simulink model "SSN_39busRT_Ctrl_4WT_19B"  (R2021a)
settings: Solver=ode3  StartTime=0.0  StopTime=10  FixedStep=Ts  MaxStep=1/60  RelTol=1e-2  AbsTol=1e-1
PreLoadFcn:
  | Ts=2.50e-6; ssn_ieee39_params; load('Pwf.mat');
InitFcn:
  | Ts=2.50e-6; ssn_ieee39_params; load('Pwf.mat');
values from neighbouring files (symbols this model uses):
  f = 50    [ssn_ieee39_params_ctrl.m]
  fNom = f    (= 60)    [ssn_ieee39_params_ctrl.m]
  ILR = 5.02    [ssn_ieee39_params_ctrl.m]
  IQMIN = 0.1    [ssn_ieee39_params_ctrl.m]
  ISCLIM = 1    [ssn_ieee39_params_ctrl.m]
  ITFpu = 1.10    (= 1.1)    [ssn_ieee39_params_ctrl.m]
  K = 1    [ssn_ieee39_params_ctrl.m]
  K1 = 1    [ssn_ieee39_params_ctrl.m]
  K2 = 2    [ssn_ieee39_params_ctrl.m]
  KCL = 1.04    [ssn_ieee39_params_ctrl.m]
  KFB = 0    [ssn_ieee39_params_ctrl.m]
  KFF = 1    [ssn_ieee39_params_ctrl.m]
  KFIX = 1    [ssn_ieee39_params_ctrl.m]
  KG = 1    [ssn_ieee39_params_ctrl.m]
  KIA = 59.91    [ssn_ieee39_params_ctrl.m]
  KIOEX = 0.0303    [ssn_ieee39_params_ctrl.m]
  KIUEX = 0.0303    [ssn_ieee39_params_ctrl.m]
  KIUOEX = 1    [ssn_ieee39_params_ctrl.m]
  KIUUEX = 1    [ssn_ieee39_params_ctrl.m]
  KLR = 22.47    [ssn_ieee39_params_ctrl.m]
  KM = 1    [ssn_ieee39_params_ctrl.m]
  KOEL = 0.24    [ssn_ieee39_params_ctrl.m]
  Kp = 1    [ssn_ieee39_params_ctrl.m]
  KPA = 30    [ssn_ieee39_params_ctrl.m]
  KPOEL = 1    [ssn_ieee39_params_ctrl.m]
  KPOEX = 0    [ssn_ieee39_params_ctrl.m]
  KPUEX = 0    [ssn_ieee39_params_ctrl.m]
  KSCALE = 0.319    [ssn_ieee39_params_ctrl.m]
  KUF = 0    [ssn_ieee39_params_ctrl.m]
  KUI = 0.001    [ssn_ieee39_params_ctrl.m]
  KUL = 0.24    [ssn_ieee39_params_ctrl.m]
  s = 10    [ssn_ieee39_params_ctrl.m]
  TA = 0.01    [ssn_ieee39_params_ctrl.m]
  Tadj = 0    [ssn_ieee39_params_ctrl.m]
  taps = [1 1 1.07 1.07 1.009 1.025 1 1.025 1.025 1.025]*1    [ssn_ieee39_params_ctrl.m]
  TF = 0.02    [ssn_ieee39_params_ctrl.m]
  TG = 0.024    [ssn_ieee39_params_ctrl.m]
  TINV = 0    [ssn_ieee39_params_ctrl.m]
  TIT = 0.1    [ssn_ieee39_params_ctrl.m]
  TL_10_11_len = 14    [ssn_ieee39_params_ctrl.m]
  TL_10_13_len = 14    [ssn_ieee39_params_ctrl.m]
  TL_13_14_len = 32    [ssn_ieee39_params_ctrl.m]
  TL_14_15_len = 70    [ssn_ieee39_params_ctrl.m]
  TL_15_16_len = 31.5    [ssn_ieee39_params_ctrl.m]
  TL_16_17_len = 26    [ssn_ieee39_params_ctrl.m]
  TL_16_19_len = 61    [ssn_ieee39_params_ctrl.m]
  TL_16_21_len = 46    [ssn_ieee39_params_ctrl.m]
  TL_16_24_len = 15    [ssn_ieee39_params_ctrl.m]
  TL_17_18_len = 26    [ssn_ieee39_params_ctrl.m]
  TL_17_27_len = 59    [ssn_ieee39_params_ctrl.m]
  TL_1_2_len = 134    [ssn_ieee39_params_ctrl.m]
  TL_1_39_len = 105    [ssn_ieee39_params_ctrl.m]
  TL_21_22_len = 47    [ssn_ieee39_params_ctrl.m]
  TL_22_23_len = 33    [ssn_ieee39_params_ctrl.m]
  TL_24_23_len = 88    [ssn_ieee39_params_ctrl.m]
  TL_25_26_len = 101    [ssn_ieee39_params_ctrl.m]
  TL_26_27_len = 46.5    [ssn_ieee39_params_ctrl.m]
  TL_26_28_len = 151    [ssn_ieee39_params_ctrl.m]
  TL_26_29_len = 200    [ssn_ieee39_params_ctrl.m]
  TL_28_29_len = 48    [ssn_ieee39_params_ctrl.m]
  TL_2_25_len = 28    [ssn_ieee39_params_ctrl.m]
  TL_2_2_len = 49    [ssn_ieee39_params_ctrl.m]
  TL_3_18_len = 42    [ssn_ieee39_params_ctrl.m]
  TL_3_4_len = 53    [ssn_ieee39_params_ctrl.m]
  TL_4_14_len = 33    [ssn_ieee39_params_ctrl.m]
  TL_4_5_len = 32.5    [ssn_ieee39_params_ctrl.m]
  TL_5_6_len = 14    [ssn_ieee39_params_ctrl.m]
  TL_5_8_len = 32    [ssn_ieee39_params_ctrl.m]
  TL_6_11_len = 26.5    [ssn_ieee39_params_ctrl.m]
  TL_6_7_len = 25.5    [ssn_ieee39_params_ctrl.m]
  TL_7_8_len = 15    [ssn_ieee39_params_ctrl.m]
  TL_8_9_len = 93    [ssn_ieee39_params_ctrl.m]
  TL_9_39_len = 136    [ssn_ieee39_params_ctrl.m]
  TOEL = 5.00    (= 5)    [ssn_ieee39_params_ctrl.m]
  TQREF = 0    [ssn_ieee39_params_ctrl.m]
  TQSCL = 0.012    [ssn_ieee39_params_ctrl.m]
  Ts_PMU = 1/1000    (= 0.001)    [ssn_ieee39_params_ctrl.m]
  TU1 = 0    [ssn_ieee39_params_ctrl.m]
  TU2 = 0    [ssn_ieee39_params_ctrl.m]
  TU3 = 0    [ssn_ieee39_params_ctrl.m]
  TU4 = 0    [ssn_ieee39_params_ctrl.m]
  TUL = 0    [ssn_ieee39_params_ctrl.m]
  TUP = 0.050    (= 0.05)    [ssn_ieee39_params_ctrl.m]
  TUQ = .005    (= 0.005)    [ssn_ieee39_params_ctrl.m]
  TUV = 0.2    [ssn_ieee39_params_ctrl.m]
  VAAMAX = VAMAX    (= 7.05)    [ssn_ieee39_params_ctrl.m]
  VAMAX = 7.05    [ssn_ieee39_params_ctrl.m]
  VAMIN = -6.11    [ssn_ieee39_params_ctrl.m]
  VBMAX = 999    [ssn_ieee39_params_ctrl.m]
  VF = 0    [ssn_ieee39_params_ctrl.m]
  VFB = 0    [ssn_ieee39_params_ctrl.m]
  VMMAX = 7.05    [ssn_ieee39_params_ctrl.m]
  VMMIN = -6.11    [ssn_ieee39_params_ctrl.m]
  VOELmax1 = 0.2353    [ssn_ieee39_params_ctrl.m]
  VOELmax2 = 0.0    (= 0)    [ssn_ieee39_params_ctrl.m]
  VOELmin1 = -0.24    [ssn_ieee39_params_ctrl.m]
  VOELmin2 = -1.0    (= -1)    [ssn_ieee39_params_ctrl.m]
  VRMAX = 7.05    [ssn_ieee39_params_ctrl.m]
  VRMIN = -6.11    [ssn_ieee39_params_ctrl.m]
  VSCLmax = 0.20    (= 0.2)    [ssn_ieee39_params_ctrl.m]
  VSCLmin = -0.10    (= -0.1)    [ssn_ieee39_params_ctrl.m]
  VUELmax1 = 1    [ssn_ieee39_params_ctrl.m]
  VUELmax2 = 1    [ssn_ieee39_params_ctrl.m]
  VUELmin1 = -1    [ssn_ieee39_params_ctrl.m]
  VUELmin2 = -1    [ssn_ieee39_params_ctrl.m]
  VUImax = 1    [ssn_ieee39_params_ctrl.m]
  VUImin = -1    [ssn_ieee39_params_ctrl.m]
undefined symbols (not defined in the file or in its folder): another_event_name, D1, Delta, DiscIntNeverNeededParam, find_system, MOV_segment9, my_event_name, powergui, Pw1, Pw2, Pw3, Pw4, vNomHV
libraries: powerlib_extras x162, spsThreePhaseVIMeasurementLib x55, spsCurrentMeasurementLib x52, simulink_extras x44, slpidlib x40, op_dpl_lib x36, spsST2AModel x20, spsThreePhaseParallelRLCLoadLib x20, spsThreePhaseTransformerTwoWindingsLib x17, spsControlledVoltageSourceLib x16, spsVoltageMeasurementLib x12, spsSynchronousMachinepuStandardLib x10
(part 19 of 19)

== system SSN_39busRT_Ctrl_4WT_19B/SM_master/4 WT/SS_windfarm1to2/Wind Farm (DFIG Type)/Wind Turbine Doubly-Fed Induction Generator (Average Model)1/Control System_average/Control/Rotor-side converter Control system/Torque control/Torque reference/Looses ==
  wr : Inport
  Idqs : Inport  Port=2
  Idq_grid_conv : Inport  Port=3
  Idqr : Inport  Port=4
  Freq : Inport  Port=5
  Constant3 : Constant  Value=R_RL
  Discrete Variable Frequency Mean value : Subsystem  mask(Discrete Variable-Frequency Mean Value){Finit=Fnom, Fmin=45, Ts=Ts_Control}
      mask prompts: Finit "Initial frequency (Hz):"; Fmin "Minimum frequency (Hz):"; Ts "Sample time:"
      mask help:
      | This discrete block computes the mean value of the input signal (port In) over a running window of one cycle of a specified frequency (port Freq).
      |
      | For the first cycle of simulation (specified by the parameter "Initial frequency"), the ouput is held to the value of the  "Initial input" parameter.
      |
      | The value of the parameter "Minimum frequency" is used to determine the buffer size of the "Variable Transport Delay" block found inside this subsystem.
      mask init:
      | MaxDelay=1/Fmin+Ts;
  Friction Factor : Gain  Gain=F  SaturateOnIntegerOverflow=on  OutDataTypeStr=Inherit: Same as input  ParamDataTypeStr=Inherit: Same as input
  Product{1..4} (4 alike) : Product  InputSameDT=on  SaturateOnIntegerOverflow=on  OutDataTypeStr=Inherit: Same as first input
  Rr : Constant  Value=Rr
  Rs : Constant  Value=Rs
  Sum2 : Sum  Inputs=+++  SaturateOnIntegerOverflow=on
  Sum5 : Sum  Inputs=|++  SaturateOnIntegerOverflow=on
  id^2+iq^2 : Fcn  Expr=u(1)^2+u(2)^2
  "id^2+iq^2 " : Fcn  Expr=u(1)^2+u(2)^2
  "id^2+iq^2   " : Fcn  Expr=u(1)^2+u(2)^2
  P_looses : Outport
  wires:
  Idqr/1 -> "id^2+iq^2 "/1
  Idqs/1 -> id^2+iq^2/1
  Discrete Variable Frequency Mean value/1(Mean) -> P_looses/1
  Sum5/1 -> Sum2/3
  Product1/1 -> Sum5/2
  Product4/1 -> Sum5/1
  Idq_grid_conv/1 -> "id^2+iq^2   "/1
  "id^2+iq^2   "/1 -> Product1/2
  Constant3/1 -> Product1/1
  wr/1 -> Product2/1, Friction Factor/1
  Sum2/1 -> Discrete Variable Frequency Mean value/2(In), Discrete Variable Frequency Mean value/3(Init)  "Looses"
  Product2/1 -> Sum2/1
  Product3/1 -> Sum2/2
  "id^2+iq^2 "/1 -> Product4/2
  Rr/1 -> Product4/1
  id^2+iq^2/1 -> Product3/2
  Rs/1 -> Product3/1
  Friction Factor/1 -> Product2/2  "T_Friction"
  Freq/1 -> Discrete Variable Frequency Mean value/1(Freq)

== system SSN_39busRT_Ctrl_4WT_19B/SM_master/4 WT/SS_windfarm1to2/Wind Farm (DFIG Type)/Wind Turbine Doubly-Fed Induction Generator (Average Model)1/Control System_average/Control/Rotor-side converter Control system/Torque control/Torque reference/Slope_B_A ==
  Constant6 : Constant  Value=power_B
  Constant7 : Constant  Value=power_A
  Constant8 : Constant  Value=speed_B
  Constant9 : Constant  Value=speed_A
  Product2 : Product  Inputs=*/  SaturateOnIntegerOverflow=on  OutDataTypeStr=Inherit: Same as first input
  Sum8 : Sum  Inputs=|+-  SaturateOnIntegerOverflow=on
  Sum9 : Sum  Inputs=|+-  SaturateOnIntegerOverflow=on
  Slope : Outport
  wires:
  Constant6/1 -> Sum8/1
  Constant7/1 -> Sum8/2
  Constant8/1 -> Sum9/1
  Constant9/1 -> Sum9/2
  Sum8/1 -> Product2/1
  Sum9/1 -> Product2/2
  Product2/1 -> Slope/1

== system SSN_39busRT_Ctrl_4WT_19B/SM_master/4 WT/SS_windfarm1to2/Wind Farm (DFIG Type)/Wind Turbine Doubly-Fed Induction Generator (Average Model)1/Control System_average/Control/Rotor-side converter Control system/Torque control/Torque reference/Slope_D_C ==
  Constant2 : Constant  Value=power_D
  Constant3 : Constant  Value=power_C
  Constant4 : Constant  Value=speed_D
  Constant5 : Constant  Value=speed_C
  Product : Product  Inputs=*/  SaturateOnIntegerOverflow=on  OutDataTypeStr=Inherit: Same as first input
  Sum6 : Sum  Inputs=|+-  SaturateOnIntegerOverflow=on
  Sum7 : Sum  Inputs=|+-  SaturateOnIntegerOverflow=on
  Slope : Outport
  wires:
  Constant2/1 -> Sum6/1
  Constant3/1 -> Sum6/2
  Constant4/1 -> Sum7/1
  Constant5/1 -> Sum7/2
  Sum6/1 -> Product/1
  Sum7/1 -> Product/2
  Product/1 -> Slope/1

== system SSN_39busRT_Ctrl_4WT_19B/SM_master/4 WT/SS_windfarm1to2/Wind Farm (DFIG Type)/Wind Turbine Doubly-Fed Induction Generator (Average Model)1/Control System_average/Control/Rotor-side converter Control system/Torque control/Torque regulator/Stator flux estimator ==
  note: Magnitude of flux at generator stator
      | The derivative components of flux are neglected
  Vdqs : Inport
  Idqs : Inport  Port=2
  Freq : Inport  Port=3
  Divide1 : Product  Inputs=*/
  Divide2 : Product  Inputs=**
  Divide3 : Product  Inputs=*/
  Divide4 : Product  Inputs=*/
  Divide6 : Product  Inputs=**
  Fnom : Constant  Value=Fnom
  Gain : Gain  Gain=-1
  Math Function1 : Math  Operator=square  SignedPower=on  SaturateOnIntegerOverflow=on
  Math Function2 : Math  Operator=square  SignedPower=on  SaturateOnIntegerOverflow=on
  Math Function3 : Math  Operator=sqrt  SignedPower=on  SaturateOnIntegerOverflow=on
  Rs : Constant  Value=Rs
  Rs2 : Constant  Value=Rs
  Selector1 : Selector  InputPortWidth=2  IndexOptions=Index vector (dialog)  Indices=2  OutputSizes=[(-2)]
  Selector2 : Selector  InputPortWidth=2  IndexOptions=Index vector (dialog)  Indices=1  OutputSizes=[(-2)]
  Selector3 : Selector  InputPortWidth=2  IndexOptions=Index vector (dialog)  Indices=2  OutputSizes=[(-2)]
  Selector4 : Selector  InputPortWidth=2  IndexOptions=Index vector (dialog)  Indices=1  OutputSizes=[(-2)]
  Sum1 : Sum  Inputs=|++
  Sum2 : Sum  Inputs=|+-
  Sum3 : Sum  Inputs=|+-
  Mag_Flux : Outport
  wires:
  Math Function2/1 -> Sum1/2
  Divide4/1 -> Math Function2/1  "phi_ds"
  Sum2/1 -> Divide4/1
  Divide2/1 -> Sum2/2  "RsIqs"
  Rs2/1 -> Divide2/2
  Selector3/1 -> Divide2/1  "Iqs"
  Selector1/1 -> Sum2/1  "Vqs"
  Math Function3/1 -> Mag_Flux/1
  Sum1/1 -> Math Function3/1
  Math Function1/1 -> Sum1/1
  Divide1/1 -> Math Function1/1  "phi_qs"
  Gain/1 -> Divide1/2
  Divide3/1 -> Divide4/2, Gain/1
  Sum3/1 -> Divide1/1
  Fnom/1 -> Divide3/2
  Freq/1 -> Divide3/1
  Selector4/1 -> Sum3/1  "Vds"
  Vdqs/1 -> Selector1/1, Selector4/1
  Rs/1 -> Divide6/2
  Selector2/1 -> Divide6/1  "Ids"
  Divide6/1 -> Sum3/2  "RsIds"
  Idqs/1 -> Selector3/1, Selector2/1

== system SSN_39busRT_Ctrl_4WT_19B/SM_master/4 WT/SS_windfarm1to2/Wind Farm (DFIG Type)1/Wind Turbine Doubly-Fed Induction Generator (Average Model)1/Control System_average/Control/Rotor-side converter Control system/Torque control/Torque reference/Looses ==
  wr : Inport
  Idqs : Inport  Port=2
  Idq_grid_conv : Inport  Port=3
  Idqr : Inport  Port=4
  Freq : Inport  Port=5
  Constant3 : Constant  Value=R_RL
  Discrete Variable Frequency Mean value : Subsystem  mask(Discrete Variable-Frequency Mean Value){Finit=Fnom, Fmin=45, Ts=Ts_Control}
      mask prompts: Finit "Initial frequency (Hz):"; Fmin "Minimum frequency (Hz):"; Ts "Sample time:"
      mask help:
      | This discrete block computes the mean value of the input signal (port In) over a running window of one cycle of a specified frequency (port Freq).
      |
      | For the first cycle of simulation (specified by the parameter "Initial frequency"), the ouput is held to the value of the  "Initial input" parameter.
      |
      | The value of the parameter "Minimum frequency" is used to determine the buffer size of the "Variable Transport Delay" block found inside this subsystem.
      mask init:
      | MaxDelay=1/Fmin+Ts;
  Friction Factor : Gain  Gain=F  SaturateOnIntegerOverflow=on  OutDataTypeStr=Inherit: Same as input  ParamDataTypeStr=Inherit: Same as input
  Product{1..4} (4 alike) : Product  InputSameDT=on  SaturateOnIntegerOverflow=on  OutDataTypeStr=Inherit: Same as first input
  Rr : Constant  Value=Rr
  Rs : Constant  Value=Rs
  Sum2 : Sum  Inputs=+++  SaturateOnIntegerOverflow=on
  Sum5 : Sum  Inputs=|++  SaturateOnIntegerOverflow=on
  id^2+iq^2 : Fcn  Expr=u(1)^2+u(2)^2
  "id^2+iq^2 " : Fcn  Expr=u(1)^2+u(2)^2
  "id^2+iq^2   " : Fcn  Expr=u(1)^2+u(2)^2
  P_looses : Outport
  wires:
  Freq/1 -> Discrete Variable Frequency Mean value/1(Freq)
  Friction Factor/1 -> Product2/2  "T_Friction"
  Rs/1 -> Product3/1
  id^2+iq^2/1 -> Product3/2
  Rr/1 -> Product4/1
  "id^2+iq^2 "/1 -> Product4/2
  Product3/1 -> Sum2/2
  Product2/1 -> Sum2/1
  Sum2/1 -> Discrete Variable Frequency Mean value/3(Init), Discrete Variable Frequency Mean value/2(In)  "Looses"
  wr/1 -> Friction Factor/1, Product2/1
  Constant3/1 -> Product1/1
  "id^2+iq^2   "/1 -> Product1/2
  Idq_grid_conv/1 -> "id^2+iq^2   "/1
  Product4/1 -> Sum5/1
  Product1/1 -> Sum5/2
  Sum5/1 -> Sum2/3
  Discrete Variable Frequency Mean value/1(Mean) -> P_looses/1
  Idqs/1 -> id^2+iq^2/1
  Idqr/1 -> "id^2+iq^2 "/1

== system SSN_39busRT_Ctrl_4WT_19B/SM_master/4 WT/SS_windfarm1to2/Wind Farm (DFIG Type)1/Wind Turbine Doubly-Fed Induction Generator (Average Model)1/Control System_average/Control/Rotor-side converter Control system/Torque control/Torque reference/Slope_B_A ==
  Constant6 : Constant  Value=power_B
  Constant7 : Constant  Value=power_A
  Constant8 : Constant  Value=speed_B
  Constant9 : Constant  Value=speed_A
  Product2 : Product  Inputs=*/  SaturateOnIntegerOverflow=on  OutDataTypeStr=Inherit: Same as first input
  Sum8 : Sum  Inputs=|+-  SaturateOnIntegerOverflow=on
  Sum9 : Sum  Inputs=|+-  SaturateOnIntegerOverflow=on
  Slope : Outport
  wires:
  Product2/1 -> Slope/1
  Sum9/1 -> Product2/2
  Sum8/1 -> Product2/1
  Constant9/1 -> Sum9/2
  Constant8/1 -> Sum9/1
  Constant7/1 -> Sum8/2
  Constant6/1 -> Sum8/1

== system SSN_39busRT_Ctrl_4WT_19B/SM_master/4 WT/SS_windfarm1to2/Wind Farm (DFIG Type)1/Wind Turbine Doubly-Fed Induction Generator (Average Model)1/Control System_average/Control/Rotor-side converter Control system/Torque control/Torque reference/Slope_D_C ==
  Constant2 : Constant  Value=power_D
  Constant3 : Constant  Value=power_C
  Constant4 : Constant  Value=speed_D
  Constant5 : Constant  Value=speed_C
  Product : Product  Inputs=*/  SaturateOnIntegerOverflow=on  OutDataTypeStr=Inherit: Same as first input
  Sum6 : Sum  Inputs=|+-  SaturateOnIntegerOverflow=on
  Sum7 : Sum  Inputs=|+-  SaturateOnIntegerOverflow=on
  Slope : Outport
  wires:
  Product/1 -> Slope/1
  Sum7/1 -> Product/2
  Sum6/1 -> Product/1
  Constant5/1 -> Sum7/2
  Constant4/1 -> Sum7/1
  Constant3/1 -> Sum6/2
  Constant2/1 -> Sum6/1

== system SSN_39busRT_Ctrl_4WT_19B/SM_master/4 WT/SS_windfarm1to2/Wind Farm (DFIG Type)1/Wind Turbine Doubly-Fed Induction Generator (Average Model)1/Control System_average/Control/Rotor-side converter Control system/Torque control/Torque regulator/Stator flux estimator ==
  note: Magnitude of flux at generator stator
      | The derivative components of flux are neglected
  Vdqs : Inport
  Idqs : Inport  Port=2
  Freq : Inport  Port=3
  Divide1 : Product  Inputs=*/
  Divide2 : Product  Inputs=**
  Divide3 : Product  Inputs=*/
  Divide4 : Product  Inputs=*/
  Divide6 : Product  Inputs=**
  Fnom : Constant  Value=Fnom
  Gain : Gain  Gain=-1
  Math Function1 : Math  Operator=square  SignedPower=on  SaturateOnIntegerOverflow=on
  Math Function2 : Math  Operator=square  SignedPower=on  SaturateOnIntegerOverflow=on
  Math Function3 : Math  Operator=sqrt  SignedPower=on  SaturateOnIntegerOverflow=on
  Rs : Constant  Value=Rs
  Rs2 : Constant  Value=Rs
  Selector1 : Selector  InputPortWidth=2  IndexOptions=Index vector (dialog)  Indices=2  OutputSizes=[(-2)]
  Selector2 : Selector  InputPortWidth=2  IndexOptions=Index vector (dialog)  Indices=1  OutputSizes=[(-2)]
  Selector3 : Selector  InputPortWidth=2  IndexOptions=Index vector (dialog)  Indices=2  OutputSizes=[(-2)]
  Selector4 : Selector  InputPortWidth=2  IndexOptions=Index vector (dialog)  Indices=1  OutputSizes=[(-2)]
  Sum1 : Sum  Inputs=|++
  Sum2 : Sum  Inputs=|+-
  Sum3 : Sum  Inputs=|+-
  Mag_Flux : Outport
  wires:
  Idqs/1 -> Selector2/1, Selector3/1
  Divide6/1 -> Sum3/2  "RsIds"
  Selector2/1 -> Divide6/1  "Ids"
  Rs/1 -> Divide6/2
  Vdqs/1 -> Selector4/1, Selector1/1
  Selector4/1 -> Sum3/1  "Vds"
  Freq/1 -> Divide3/1
  Fnom/1 -> Divide3/2
  Sum3/1 -> Divide1/1
  Divide3/1 -> Gain/1, Divide4/2
  Gain/1 -> Divide1/2
  Divide1/1 -> Math Function1/1  "phi_qs"
  Math Function1/1 -> Sum1/1
  Sum1/1 -> Math Function3/1
  Math Function3/1 -> Mag_Flux/1
  Selector1/1 -> Sum2/1  "Vqs"
  Selector3/1 -> Divide2/1  "Iqs"
  Rs2/1 -> Divide2/2
  Divide2/1 -> Sum2/2  "RsIqs"
  Sum2/1 -> Divide4/1
  Divide4/1 -> Math Function2/1  "phi_ds"
  Math Function2/1 -> Sum1/2

== system SSN_39busRT_Ctrl_4WT_19B/SM_master/4 WT/SS_windfarm3to4/Wind Farm (DFIG Type)/Wind Turbine Doubly-Fed Induction Generator (Average Model)1/Control System_average/Control/Rotor-side converter Control system/Torque control/Torque reference/Looses ==
  wr : Inport
  Idqs : Inport  Port=2
  Idq_grid_conv : Inport  Port=3
  Idqr : Inport  Port=4
  Freq : Inport  Port=5
  Constant3 : Constant  Value=R_RL
  Discrete Variable Frequency Mean value : Subsystem  mask(Discrete Variable-Frequency Mean Value){Finit=Fnom, Fmin=45, Ts=Ts_Control}
      mask prompts: Finit "Initial frequency (Hz):"; Fmin "Minimum frequency (Hz):"; Ts "Sample time:"
      mask help:
      | This discrete block computes the mean value of the input signal (port In) over a running window of one cycle of a specified frequency (port Freq).
      |
      | For the first cycle of simulation (specified by the parameter "Initial frequency"), the ouput is held to the value of the  "Initial input" parameter.
      |
      | The value of the parameter "Minimum frequency" is used to determine the buffer size of the "Variable Transport Delay" block found inside this subsystem.
      mask init:
      | MaxDelay=1/Fmin+Ts;
  Friction Factor : Gain  Gain=F  SaturateOnIntegerOverflow=on  OutDataTypeStr=Inherit: Same as input  ParamDataTypeStr=Inherit: Same as input
  Product{1..4} (4 alike) : Product  InputSameDT=on  SaturateOnIntegerOverflow=on  OutDataTypeStr=Inherit: Same as first input
  Rr : Constant  Value=Rr
  Rs : Constant  Value=Rs
  Sum2 : Sum  Inputs=+++  SaturateOnIntegerOverflow=on
  Sum5 : Sum  Inputs=|++  SaturateOnIntegerOverflow=on
  id^2+iq^2 : Fcn  Expr=u(1)^2+u(2)^2
  "id^2+iq^2 " : Fcn  Expr=u(1)^2+u(2)^2
  "id^2+iq^2   " : Fcn  Expr=u(1)^2+u(2)^2
  P_looses : Outport
  wires:
  Idqr/1 -> "id^2+iq^2 "/1
  Idqs/1 -> id^2+iq^2/1
  Discrete Variable Frequency Mean value/1(Mean) -> P_looses/1
  Sum5/1 -> Sum2/3
  Product1/1 -> Sum5/2
  Product4/1 -> Sum5/1
  Idq_grid_conv/1 -> "id^2+iq^2   "/1
  "id^2+iq^2   "/1 -> Product1/2
  Constant3/1 -> Product1/1
  wr/1 -> Product2/1, Friction Factor/1
  Sum2/1 -> Discrete Variable Frequency Mean value/2(In), Discrete Variable Frequency Mean value/3(Init)  "Looses"
  Product2/1 -> Sum2/1
  Product3/1 -> Sum2/2
  "id^2+iq^2 "/1 -> Product4/2
  Rr/1 -> Product4/1
  id^2+iq^2/1 -> Product3/2
  Rs/1 -> Product3/1
  Friction Factor/1 -> Product2/2  "T_Friction"
  Freq/1 -> Discrete Variable Frequency Mean value/1(Freq)

== system SSN_39busRT_Ctrl_4WT_19B/SM_master/4 WT/SS_windfarm3to4/Wind Farm (DFIG Type)/Wind Turbine Doubly-Fed Induction Generator (Average Model)1/Control System_average/Control/Rotor-side converter Control system/Torque control/Torque reference/Slope_B_A ==
  Constant6 : Constant  Value=power_B
  Constant7 : Constant  Value=power_A
  Constant8 : Constant  Value=speed_B
  Constant9 : Constant  Value=speed_A
  Product2 : Product  Inputs=*/  SaturateOnIntegerOverflow=on  OutDataTypeStr=Inherit: Same as first input
  Sum8 : Sum  Inputs=|+-  SaturateOnIntegerOverflow=on
  Sum9 : Sum  Inputs=|+-  SaturateOnIntegerOverflow=on
  Slope : Outport
  wires:
  Constant6/1 -> Sum8/1
  Constant7/1 -> Sum8/2
  Constant8/1 -> Sum9/1
  Constant9/1 -> Sum9/2
  Sum8/1 -> Product2/1
  Sum9/1 -> Product2/2
  Product2/1 -> Slope/1

== system SSN_39busRT_Ctrl_4WT_19B/SM_master/4 WT/SS_windfarm3to4/Wind Farm (DFIG Type)/Wind Turbine Doubly-Fed Induction Generator (Average Model)1/Control System_average/Control/Rotor-side converter Control system/Torque control/Torque reference/Slope_D_C ==
  Constant2 : Constant  Value=power_D
  Constant3 : Constant  Value=power_C
  Constant4 : Constant  Value=speed_D
  Constant5 : Constant  Value=speed_C
  Product : Product  Inputs=*/  SaturateOnIntegerOverflow=on  OutDataTypeStr=Inherit: Same as first input
  Sum6 : Sum  Inputs=|+-  SaturateOnIntegerOverflow=on
  Sum7 : Sum  Inputs=|+-  SaturateOnIntegerOverflow=on
  Slope : Outport
  wires:
  Constant2/1 -> Sum6/1
  Constant3/1 -> Sum6/2
  Constant4/1 -> Sum7/1
  Constant5/1 -> Sum7/2
  Sum6/1 -> Product/1
  Sum7/1 -> Product/2
  Product/1 -> Slope/1

== system SSN_39busRT_Ctrl_4WT_19B/SM_master/4 WT/SS_windfarm3to4/Wind Farm (DFIG Type)/Wind Turbine Doubly-Fed Induction Generator (Average Model)1/Control System_average/Control/Rotor-side converter Control system/Torque control/Torque regulator/Stator flux estimator ==
  note: Magnitude of flux at generator stator
      | The derivative components of flux are neglected
  Vdqs : Inport
  Idqs : Inport  Port=2
  Freq : Inport  Port=3
  Divide1 : Product  Inputs=*/
  Divide2 : Product  Inputs=**
  Divide3 : Product  Inputs=*/
  Divide4 : Product  Inputs=*/
  Divide6 : Product  Inputs=**
  Fnom : Constant  Value=Fnom
  Gain : Gain  Gain=-1
  Math Function1 : Math  Operator=square  SignedPower=on  SaturateOnIntegerOverflow=on
  Math Function2 : Math  Operator=square  SignedPower=on  SaturateOnIntegerOverflow=on
  Math Function3 : Math  Operator=sqrt  SignedPower=on  SaturateOnIntegerOverflow=on
  Rs : Constant  Value=Rs
  Rs2 : Constant  Value=Rs
  Selector1 : Selector  InputPortWidth=2  IndexOptions=Index vector (dialog)  Indices=2  OutputSizes=[(-2)]
  Selector2 : Selector  InputPortWidth=2  IndexOptions=Index vector (dialog)  Indices=1  OutputSizes=[(-2)]
  Selector3 : Selector  InputPortWidth=2  IndexOptions=Index vector (dialog)  Indices=2  OutputSizes=[(-2)]
  Selector4 : Selector  InputPortWidth=2  IndexOptions=Index vector (dialog)  Indices=1  OutputSizes=[(-2)]
  Sum1 : Sum  Inputs=|++
  Sum2 : Sum  Inputs=|+-
  Sum3 : Sum  Inputs=|+-
  Mag_Flux : Outport
  wires:
  Math Function2/1 -> Sum1/2
  Divide4/1 -> Math Function2/1  "phi_ds"
  Sum2/1 -> Divide4/1
  Divide2/1 -> Sum2/2  "RsIqs"
  Rs2/1 -> Divide2/2
  Selector3/1 -> Divide2/1  "Iqs"
  Selector1/1 -> Sum2/1  "Vqs"
  Math Function3/1 -> Mag_Flux/1
  Sum1/1 -> Math Function3/1
  Math Function1/1 -> Sum1/1
  Divide1/1 -> Math Function1/1  "phi_qs"
  Gain/1 -> Divide1/2
  Divide3/1 -> Divide4/2, Gain/1
  Sum3/1 -> Divide1/1
  Fnom/1 -> Divide3/2
  Freq/1 -> Divide3/1
  Selector4/1 -> Sum3/1  "Vds"
  Vdqs/1 -> Selector1/1, Selector4/1
  Rs/1 -> Divide6/2
  Selector2/1 -> Divide6/1  "Ids"
  Divide6/1 -> Sum3/2  "RsIds"
  Idqs/1 -> Selector3/1, Selector2/1

== system SSN_39busRT_Ctrl_4WT_19B/SM_master/4 WT/SS_windfarm3to4/Wind Farm (DFIG Type)2/Wind Turbine Doubly-Fed Induction Generator (Average Model)1/Control System_average/Control/Rotor-side converter Control system/Torque control/Torque reference/Looses ==
  wr : Inport
  Idqs : Inport  Port=2
  Idq_grid_conv : Inport  Port=3
  Idqr : Inport  Port=4
  Freq : Inport  Port=5
  Constant3 : Constant  Value=R_RL
  Discrete Variable Frequency Mean value : Subsystem  mask(Discrete Variable-Frequency Mean Value){Finit=Fnom, Fmin=45, Ts=Ts_Control}
      mask prompts: Finit "Initial frequency (Hz):"; Fmin "Minimum frequency (Hz):"; Ts "Sample time:"
      mask help:
      | This discrete block computes the mean value of the input signal (port In) over a running window of one cycle of a specified frequency (port Freq).
      |
      | For the first cycle of simulation (specified by the parameter "Initial frequency"), the ouput is held to the value of the  "Initial input" parameter.
      |
      | The value of the parameter "Minimum frequency" is used to determine the buffer size of the "Variable Transport Delay" block found inside this subsystem.
      mask init:
      | MaxDelay=1/Fmin+Ts;
  Friction Factor : Gain  Gain=F  SaturateOnIntegerOverflow=on  OutDataTypeStr=Inherit: Same as input  ParamDataTypeStr=Inherit: Same as input
  Product{1..4} (4 alike) : Product  InputSameDT=on  SaturateOnIntegerOverflow=on  OutDataTypeStr=Inherit: Same as first input
  Rr : Constant  Value=Rr
  Rs : Constant  Value=Rs
  Sum2 : Sum  Inputs=+++  SaturateOnIntegerOverflow=on
  Sum5 : Sum  Inputs=|++  SaturateOnIntegerOverflow=on
  id^2+iq^2 : Fcn  Expr=u(1)^2+u(2)^2
  "id^2+iq^2 " : Fcn  Expr=u(1)^2+u(2)^2
  "id^2+iq^2   " : Fcn  Expr=u(1)^2+u(2)^2
  P_looses : Outport
  wires:
  Freq/1 -> Discrete Variable Frequency Mean value/1(Freq)
  Friction Factor/1 -> Product2/2  "T_Friction"
  Rs/1 -> Product3/1
  id^2+iq^2/1 -> Product3/2
  Rr/1 -> Product4/1
  "id^2+iq^2 "/1 -> Product4/2
  Product3/1 -> Sum2/2
  Product2/1 -> Sum2/1
  Sum2/1 -> Discrete Variable Frequency Mean value/3(Init), Discrete Variable Frequency Mean value/2(In)  "Looses"
  wr/1 -> Friction Factor/1, Product2/1
  Constant3/1 -> Product1/1
  "id^2+iq^2   "/1 -> Product1/2
  Idq_grid_conv/1 -> "id^2+iq^2   "/1
  Product4/1 -> Sum5/1
  Product1/1 -> Sum5/2
  Sum5/1 -> Sum2/3
  Discrete Variable Frequency Mean value/1(Mean) -> P_looses/1
  Idqs/1 -> id^2+iq^2/1
  Idqr/1 -> "id^2+iq^2 "/1

== system SSN_39busRT_Ctrl_4WT_19B/SM_master/4 WT/SS_windfarm3to4/Wind Farm (DFIG Type)2/Wind Turbine Doubly-Fed Induction Generator (Average Model)1/Control System_average/Control/Rotor-side converter Control system/Torque control/Torque reference/Slope_B_A ==
  Constant6 : Constant  Value=power_B
  Constant7 : Constant  Value=power_A
  Constant8 : Constant  Value=speed_B
  Constant9 : Constant  Value=speed_A
  Product2 : Product  Inputs=*/  SaturateOnIntegerOverflow=on  OutDataTypeStr=Inherit: Same as first input
  Sum8 : Sum  Inputs=|+-  SaturateOnIntegerOverflow=on
  Sum9 : Sum  Inputs=|+-  SaturateOnIntegerOverflow=on
  Slope : Outport
  wires:
  Product2/1 -> Slope/1
  Sum9/1 -> Product2/2
  Sum8/1 -> Product2/1
  Constant9/1 -> Sum9/2
  Constant8/1 -> Sum9/1
  Constant7/1 -> Sum8/2
  Constant6/1 -> Sum8/1

== system SSN_39busRT_Ctrl_4WT_19B/SM_master/4 WT/SS_windfarm3to4/Wind Farm (DFIG Type)2/Wind Turbine Doubly-Fed Induction Generator (Average Model)1/Control System_average/Control/Rotor-side converter Control system/Torque control/Torque reference/Slope_D_C ==
  Constant2 : Constant  Value=power_D
  Constant3 : Constant  Value=power_C
  Constant4 : Constant  Value=speed_D
  Constant5 : Constant  Value=speed_C
  Product : Product  Inputs=*/  SaturateOnIntegerOverflow=on  OutDataTypeStr=Inherit: Same as first input
  Sum6 : Sum  Inputs=|+-  SaturateOnIntegerOverflow=on
  Sum7 : Sum  Inputs=|+-  SaturateOnIntegerOverflow=on
  Slope : Outport
  wires:
  Product/1 -> Slope/1
  Sum7/1 -> Product/2
  Sum6/1 -> Product/1
  Constant5/1 -> Sum7/2
  Constant4/1 -> Sum7/1
  Constant3/1 -> Sum6/2
  Constant2/1 -> Sum6/1

== system SSN_39busRT_Ctrl_4WT_19B/SM_master/4 WT/SS_windfarm3to4/Wind Farm (DFIG Type)2/Wind Turbine Doubly-Fed Induction Generator (Average Model)1/Control System_average/Control/Rotor-side converter Control system/Torque control/Torque regulator/Stator flux estimator ==
  note: Magnitude of flux at generator stator
      | The derivative components of flux are neglected
  Vdqs : Inport
  Idqs : Inport  Port=2
  Freq : Inport  Port=3
  Divide1 : Product  Inputs=*/
  Divide2 : Product  Inputs=**
  Divide3 : Product  Inputs=*/
  Divide4 : Product  Inputs=*/
  Divide6 : Product  Inputs=**
  Fnom : Constant  Value=Fnom
  Gain : Gain  Gain=-1
  Math Function1 : Math  Operator=square  SignedPower=on  SaturateOnIntegerOverflow=on
  Math Function2 : Math  Operator=square  SignedPower=on  SaturateOnIntegerOverflow=on
  Math Function3 : Math  Operator=sqrt  SignedPower=on  SaturateOnIntegerOverflow=on
  Rs : Constant  Value=Rs
  Rs2 : Constant  Value=Rs
  Selector1 : Selector  InputPortWidth=2  IndexOptions=Index vector (dialog)  Indices=2  OutputSizes=[(-2)]
  Selector2 : Selector  InputPortWidth=2  IndexOptions=Index vector (dialog)  Indices=1  OutputSizes=[(-2)]
  Selector3 : Selector  InputPortWidth=2  IndexOptions=Index vector (dialog)  Indices=2  OutputSizes=[(-2)]
  Selector4 : Selector  InputPortWidth=2  IndexOptions=Index vector (dialog)  Indices=1  OutputSizes=[(-2)]
  Sum1 : Sum  Inputs=|++
  Sum2 : Sum  Inputs=|+-
  Sum3 : Sum  Inputs=|+-
  Mag_Flux : Outport
  wires:
  Idqs/1 -> Selector2/1, Selector3/1
  Divide6/1 -> Sum3/2  "RsIds"
  Selector2/1 -> Divide6/1  "Ids"
  Rs/1 -> Divide6/2
  Vdqs/1 -> Selector4/1, Selector1/1
  Selector4/1 -> Sum3/1  "Vds"
  Freq/1 -> Divide3/1
  Fnom/1 -> Divide3/2
  Sum3/1 -> Divide1/1
  Divide3/1 -> Gain/1, Divide4/2
  Gain/1 -> Divide1/2
  Divide1/1 -> Math Function1/1  "phi_qs"
  Math Function1/1 -> Sum1/1
  Sum1/1 -> Math Function3/1
  Math Function3/1 -> Mag_Flux/1
  Selector1/1 -> Sum2/1  "Vqs"
  Selector3/1 -> Divide2/1  "Iqs"
  Rs2/1 -> Divide2/2
  Divide2/1 -> Sum2/2  "RsIqs"
  Sum2/1 -> Divide4/1
  Divide4/1 -> Math Function2/1  "phi_ds"
  Math Function2/1 -> Sum1/2

== system SSN_39busRT_Ctrl_4WT_19B/SM_master/4 WT/SS_windfarm1to2/Wind Farm (DFIG Type)/Wind Turbine Doubly-Fed Induction Generator (Average Model)1/Control System_average/Control/Rotor-side converter Control system/Torque control/Torque reference/Looses/Discrete Variable Frequency Mean value ==
  note: Variable frequency - Discrete Mean Value
  note: Pierre Giroux, Gilbert Sybille, Richard Gagnon
      | Power System Simulation Laboratory
      | IREQ, Hydro-Quebc
  note: link disabled
  Freq : Inport  PortDimensions=1
  In : Inport  Port=2  PortDimensions=1
  Init : Inport  Port=3
  Correction subsystem : powerlib_extras/Discrete Measurements/Discrete Variable Frequency Mean value/Correction subsystem  SystemSampleTime=-1  VariantActivationTime=update diagram  Latency=0  AutoFrameSizeCalculation=off
      settings: SourceProductBaseCode=PS
  Discrete Variable Transport Delay : powerlib_extras/Discrete  Control Blocks/Discrete Variable Transport Delay  MaxDelay=MaxDelay  InitialValue=0  Ts=Ts
      settings: SourceProductBaseCode=PS
  Gain : Gain  Gain=Ts  SaturateOnIntegerOverflow=on  OutDataTypeStr=Inherit: Same as input  ParamDataTypeStr=Inherit: Same as input
  Integ4 : DiscreteIntegrator  IntegratorMethod=Integration: Trapezoidal  SampleTime=Ts  ICPrevOutput=DiscIntNeverNeededParam  ICPrevScaledInput=DiscIntNeverNeededParam
  Number of samples per cycle : Fcn  Expr=1/u[1]/Ts
  Product : Product  InputSameDT=on  SaturateOnIntegerOverflow=on  OutDataTypeStr=Inherit: Same as first input
  Rounding Function : Rounding  Operator=ceil
  Step : Step  Time=1/Finit  SampleTime=Ts
  Sum5 : Sum  InputSameDT=on  SaturateOnIntegerOverflow=on  OutDataTypeStr=Inherit: Same as first input
  Sum7 : Sum  Inputs=-+  InputSameDT=on  SaturateOnIntegerOverflow=on  OutDataTypeStr=Inherit: Same as first input
  Switch : Switch  Threshold=0.5  InputSameDT=on
  To avoid division by zero : Saturate  UpperLimit=1e6  LowerLimit=1e-6
  Mean : Outport
  wires:
  Step/1 -> Switch/2
  Correction subsystem/1 -> Sum5/2
  To avoid division by zero/1 -> Number of samples per cycle/1  "Freq"
  Switch/1 -> Mean/1
  Init/1 -> Switch/3
  Sum5/1 -> Switch/1
  Number of samples per cycle/1 -> Correction subsystem/1, Rounding Function/1
  Rounding Function/1 -> Correction subsystem/2, Gain/1
  Gain/1 -> Discrete Variable Transport Delay/2  "Delay"
  Freq/1 -> To avoid division by zero/1, Product/2  "Freq"
  Integ4/1 -> Sum7/2, Discrete Variable Transport Delay/1
  Sum7/1 -> Product/1
  Discrete Variable Transport Delay/1 -> Sum7/1
  Product/1 -> Sum5/1  "Mean value"
  In/1 -> Correction subsystem/3, Integ4/1  "In"

== system SSN_39busRT_Ctrl_4WT_19B/SM_master/4 WT/SS_windfarm1to2/Wind Farm (DFIG Type)1/Wind Turbine Doubly-Fed Induction Generator (Average Model)1/Control System_average/Control/Rotor-side converter Control system/Torque control/Torque reference/Looses/Discrete Variable Frequency Mean value ==
  note: link disabled
  note: Pierre Giroux, Gilbert Sybille, Richard Gagnon
      | Power System Simulation Laboratory
      | IREQ, Hydro-Quebc
  note: Variable frequency - Discrete Mean Value
  Freq : Inport  PortDimensions=1
  In : Inport  Port=2  PortDimensions=1
  Init : Inport  Port=3
  Correction subsystem : powerlib_extras/Discrete Measurements/Discrete Variable Frequency Mean value/Correction subsystem  SystemSampleTime=-1  VariantActivationTime=update diagram  Latency=0  AutoFrameSizeCalculation=off
      settings: SourceProductBaseCode=PS
  Discrete Variable Transport Delay : powerlib_extras/Discrete  Control Blocks/Discrete Variable Transport Delay  MaxDelay=MaxDelay  InitialValue=0  Ts=Ts
      settings: SourceProductBaseCode=PS
  Gain : Gain  Gain=Ts  SaturateOnIntegerOverflow=on  OutDataTypeStr=Inherit: Same as input  ParamDataTypeStr=Inherit: Same as input
  Integ4 : DiscreteIntegrator  IntegratorMethod=Integration: Trapezoidal  SampleTime=Ts  ICPrevOutput=DiscIntNeverNeededParam  ICPrevScaledInput=DiscIntNeverNeededParam
  Number of samples per cycle : Fcn  Expr=1/u[1]/Ts
  Product : Product  InputSameDT=on  SaturateOnIntegerOverflow=on  OutDataTypeStr=Inherit: Same as first input
  Rounding Function : Rounding  Operator=ceil
  Step : Step  Time=1/Finit  SampleTime=Ts
  Sum5 : Sum  InputSameDT=on  SaturateOnIntegerOverflow=on  OutDataTypeStr=Inherit: Same as first input
  Sum7 : Sum  Inputs=-+  InputSameDT=on  SaturateOnIntegerOverflow=on  OutDataTypeStr=Inherit: Same as first input
  Switch : Switch  Threshold=0.5  InputSameDT=on
  To avoid division by zero : Saturate  UpperLimit=1e6  LowerLimit=1e-6
  Mean : Outport
  wires:
  In/1 -> Integ4/1, Correction subsystem/3  "In"
  Product/1 -> Sum5/1  "Mean value"
  Discrete Variable Transport Delay/1 -> Sum7/1
  Sum7/1 -> Product/1
  Integ4/1 -> Discrete Variable Transport Delay/1, Sum7/2
  Freq/1 -> Product/2, To avoid division by zero/1  "Freq"
  Gain/1 -> Discrete Variable Transport Delay/2  "Delay"
  Rounding Function/1 -> Gain/1, Correction subsystem/2
  Number of samples per cycle/1 -> Rounding Function/1, Correction subsystem/1
  Sum5/1 -> Switch/1
  Init/1 -> Switch/3
  Switch/1 -> Mean/1
  To avoid division by zero/1 -> Number of samples per cycle/1  "Freq"
  Correction subsystem/1 -> Sum5/2
  Step/1 -> Switch/2

== system SSN_39busRT_Ctrl_4WT_19B/SM_master/4 WT/SS_windfarm3to4/Wind Farm (DFIG Type)/Wind Turbine Doubly-Fed Induction Generator (Average Model)1/Control System_average/Control/Rotor-side converter Control system/Torque control/Torque reference/Looses/Discrete Variable Frequency Mean value ==
  note: Variable frequency - Discrete Mean Value
  note: Pierre Giroux, Gilbert Sybille, Richard Gagnon
      | Power System Simulation Laboratory
      | IREQ, Hydro-Quebc
  note: link disabled
  Freq : Inport  PortDimensions=1
  In : Inport  Port=2  PortDimensions=1
  Init : Inport  Port=3
  Correction subsystem : powerlib_extras/Discrete Measurements/Discrete Variable Frequency Mean value/Correction subsystem  SystemSampleTime=-1  VariantActivationTime=update diagram  Latency=0  AutoFrameSizeCalculation=off
      settings: SourceProductBaseCode=PS
  Discrete Variable Transport Delay : powerlib_extras/Discrete  Control Blocks/Discrete Variable Transport Delay  MaxDelay=MaxDelay  InitialValue=0  Ts=Ts
      settings: SourceProductBaseCode=PS
  Gain : Gain  Gain=Ts  SaturateOnIntegerOverflow=on  OutDataTypeStr=Inherit: Same as input  ParamDataTypeStr=Inherit: Same as input
  Integ4 : DiscreteIntegrator  IntegratorMethod=Integration: Trapezoidal  SampleTime=Ts  ICPrevOutput=DiscIntNeverNeededParam  ICPrevScaledInput=DiscIntNeverNeededParam
  Number of samples per cycle : Fcn  Expr=1/u[1]/Ts
  Product : Product  InputSameDT=on  SaturateOnIntegerOverflow=on  OutDataTypeStr=Inherit: Same as first input
  Rounding Function : Rounding  Operator=ceil
  Step : Step  Time=1/Finit  SampleTime=Ts
  Sum5 : Sum  InputSameDT=on  SaturateOnIntegerOverflow=on  OutDataTypeStr=Inherit: Same as first input
  Sum7 : Sum  Inputs=-+  InputSameDT=on  SaturateOnIntegerOverflow=on  OutDataTypeStr=Inherit: Same as first input
  Switch : Switch  Threshold=0.5  InputSameDT=on
  To avoid division by zero : Saturate  UpperLimit=1e6  LowerLimit=1e-6
  Mean : Outport
  wires:
  Step/1 -> Switch/2
  Correction subsystem/1 -> Sum5/2
  To avoid division by zero/1 -> Number of samples per cycle/1  "Freq"
  Switch/1 -> Mean/1
  Init/1 -> Switch/3
  Sum5/1 -> Switch/1
  Number of samples per cycle/1 -> Correction subsystem/1, Rounding Function/1
  Rounding Function/1 -> Correction subsystem/2, Gain/1
  Gain/1 -> Discrete Variable Transport Delay/2  "Delay"
  Freq/1 -> To avoid division by zero/1, Product/2  "Freq"
  Integ4/1 -> Sum7/2, Discrete Variable Transport Delay/1
  Sum7/1 -> Product/1
  Discrete Variable Transport Delay/1 -> Sum7/1
  Product/1 -> Sum5/1  "Mean value"
  In/1 -> Correction subsystem/3, Integ4/1  "In"

== system SSN_39busRT_Ctrl_4WT_19B/SM_master/4 WT/SS_windfarm3to4/Wind Farm (DFIG Type)2/Wind Turbine Doubly-Fed Induction Generator (Average Model)1/Control System_average/Control/Rotor-side converter Control system/Torque control/Torque reference/Looses/Discrete Variable Frequency Mean value ==
  note: link disabled
  note: Pierre Giroux, Gilbert Sybille, Richard Gagnon
      | Power System Simulation Laboratory
      | IREQ, Hydro-Quebc
  note: Variable frequency - Discrete Mean Value
  Freq : Inport  PortDimensions=1
  In : Inport  Port=2  PortDimensions=1
  Init : Inport  Port=3
  Correction subsystem : powerlib_extras/Discrete Measurements/Discrete Variable Frequency Mean value/Correction subsystem  SystemSampleTime=-1  VariantActivationTime=update diagram  Latency=0  AutoFrameSizeCalculation=off
      settings: SourceProductBaseCode=PS
  Discrete Variable Transport Delay : powerlib_extras/Discrete  Control Blocks/Discrete Variable Transport Delay  MaxDelay=MaxDelay  InitialValue=0  Ts=Ts
      settings: SourceProductBaseCode=PS
  Gain : Gain  Gain=Ts  SaturateOnIntegerOverflow=on  OutDataTypeStr=Inherit: Same as input  ParamDataTypeStr=Inherit: Same as input
  Integ4 : DiscreteIntegrator  IntegratorMethod=Integration: Trapezoidal  SampleTime=Ts  ICPrevOutput=DiscIntNeverNeededParam  ICPrevScaledInput=DiscIntNeverNeededParam
  Number of samples per cycle : Fcn  Expr=1/u[1]/Ts
  Product : Product  InputSameDT=on  SaturateOnIntegerOverflow=on  OutDataTypeStr=Inherit: Same as first input
  Rounding Function : Rounding  Operator=ceil
  Step : Step  Time=1/Finit  SampleTime=Ts
  Sum5 : Sum  InputSameDT=on  SaturateOnIntegerOverflow=on  OutDataTypeStr=Inherit: Same as first input
  Sum7 : Sum  Inputs=-+  InputSameDT=on  SaturateOnIntegerOverflow=on  OutDataTypeStr=Inherit: Same as first input
  Switch : Switch  Threshold=0.5  InputSameDT=on
  To avoid division by zero : Saturate  UpperLimit=1e6  LowerLimit=1e-6
  Mean : Outport
  wires:
  In/1 -> Integ4/1, Correction subsystem/3  "In"
  Product/1 -> Sum5/1  "Mean value"
  Discrete Variable Transport Delay/1 -> Sum7/1
  Sum7/1 -> Product/1
  Integ4/1 -> Discrete Variable Transport Delay/1, Sum7/2
  Freq/1 -> Product/2, To avoid division by zero/1  "Freq"
  Gain/1 -> Discrete Variable Transport Delay/2  "Delay"
  Rounding Function/1 -> Gain/1, Correction subsystem/2
  Number of samples per cycle/1 -> Rounding Function/1, Correction subsystem/1
  Sum5/1 -> Switch/1
  Init/1 -> Switch/3
  Switch/1 -> Mean/1
  To avoid division by zero/1 -> Number of samples per cycle/1  "Freq"
  Correction subsystem/1 -> Sum5/2
  Step/1 -> Switch/2

== matlab function SSN_39busRT_Ctrl_4WT_19B/SM_master/G10/G10/ST6C EXCITER-1/MATLAB Function ==
  data: VTF input; u output; Vbias input
function u = fcn(VTF,Vbias)
%#codegen
if VTF > 1
    u=VTF;
    
else if VTF > Vbias
        u=1;
    else
        u=VTF/Vbias
    end
end
u;

== matlab function SSN_39busRT_Ctrl_4WT_19B/SM_master/G8/ G8/ST6C EXCITER-1/MATLAB Function1 ==
  data: VT input; u output; QT input; PT input
function u = fcn(VT,QT,PT)
Xq=0.474;
Kadj= (((VT*VT)/Xq)+QT)/(sqrt(((((VT*VT)/Xq)+QT)*(((VT*VT)/Xq)+QT))+(PT*PT)))
u= Kadj;

== matlab function SSN_39busRT_Ctrl_4WT_19B/SM_master/G8/ G8/ST6C EXCITER-1/MATLAB Function2 ==
  data: ISCLERR input; IOEX2 output; ISCLINV input; IUEX2 output
function [IOEX2,IUEX2] = fcn(ISCLERR,ISCLINV)
%#codegen

IOEX2= 0;
IUEX2= 0;

== matlab function SSN_39busRT_Ctrl_4WT_19B/SM_master/G2/G2/ST6C EXCITER-1/MATLAB Function1 ==
  data: VT input; u output; QT input; PT input
function u = fcn(VT,QT,PT)
Xq=0.474;
Kadj= (((VT*VT)/Xq)+QT)/(sqrt(((((VT*VT)/Xq)+QT)*(((VT*VT)/Xq)+QT))+(PT*PT)))
u= Kadj;

== matlab function SSN_39busRT_Ctrl_4WT_19B/SM_master/G2/G2/ST6C EXCITER-1/MATLAB Function2 ==
  data: ISCLERR input; IOEX2 output; ISCLINV input; IUEX2 output
function [IOEX2,IUEX2] = fcn(ISCLERR,ISCLINV)
%#codegen

IOEX2= 0;
IUEX2= 0;

== matlab function SSN_39busRT_Ctrl_4WT_19B/SM_master/G6/G6/ST6C EXCITER-1/MATLAB Function ==
  data: VTF input; u output; Vbias input
function u = fcn(VTF,Vbias)
%#codegen
if VTF > 1
    u=VTF;
    
else if VTF > Vbias
        u=1;
    else
        u=VTF/Vbias
    end
end
u;

== matlab function SSN_39busRT_Ctrl_4WT_19B/SM_master/G6/G6/ST6C EXCITER-1/MATLAB Function1 ==
  data: VT input; u output; QT input; PT input
function u = fcn(VT,QT,PT)
Xq=0.474;
Kadj= (((VT*VT)/Xq)+QT)/(sqrt(((((VT*VT)/Xq)+QT)*(((VT*VT)/Xq)+QT))+(PT*PT)))
u= Kadj;

== matlab function SSN_39busRT_Ctrl_4WT_19B/SM_master/G6/G6/ST6C EXCITER-1/MATLAB Function2 ==
  data: ISCLERR input; IOEX2 output; ISCLINV input; IUEX2 output
function [IOEX2,IUEX2] = fcn(ISCLERR,ISCLINV)
%#codegen

IOEX2= 0;
IUEX2= 0;

== matlab function SSN_39busRT_Ctrl_4WT_19B/SM_master/G5/G5/ST6C EXCITER-1/MATLAB Function ==
  data: VTF input; u output; Vbias input
function u = fcn(VTF,Vbias)
%#codegen
if VTF > 1
    u=VTF;
    
else if VTF > Vbias
        u=1;
    else
        u=VTF/Vbias
    end
end
u;

== matlab function SSN_39busRT_Ctrl_4WT_19B/SM_master/G5/G5/ST6C EXCITER-1/MATLAB Function1 ==
  data: VT input; u output; QT input; PT input
function u = fcn(VT,QT,PT)
Xq=0.474;
Kadj= (((VT*VT)/Xq)+QT)/(sqrt(((((VT*VT)/Xq)+QT)*(((VT*VT)/Xq)+QT))+(PT*PT)))
u= Kadj;

== matlab function SSN_39busRT_Ctrl_4WT_19B/SM_master/G10/G10/ST6C EXCITER-1/MATLAB Function1 ==
  data: VT input; u output; QT input; PT input
function u = fcn(VT,QT,PT)
Xq=0.474;
Kadj= (((VT*VT)/Xq)+QT)/(sqrt(((((VT*VT)/Xq)+QT)*(((VT*VT)/Xq)+QT))+(PT*PT)))
u= Kadj;

== matlab function SSN_39busRT_Ctrl_4WT_19B/SM_master/G5/G5/ST6C EXCITER-1/MATLAB Function2 ==
  data: ISCLERR input; IOEX2 output; ISCLINV input; IUEX2 output
function [IOEX2,IUEX2] = fcn(ISCLERR,ISCLINV)
%#codegen

IOEX2= 0;
IUEX2= 0;

== matlab function SSN_39busRT_Ctrl_4WT_19B/SM_master/G4/G4/ST6C EXCITER-1/MATLAB Function ==
  data: VTF input; u output; Vbias input
function u = fcn(VTF,Vbias)
%#codegen
if VTF > 1
    u=VTF;
    
else if VTF > Vbias
        u=1;
    else
        u=VTF/Vbias
    end
end
u;

== matlab function SSN_39busRT_Ctrl_4WT_19B/SM_master/G4/G4/ST6C EXCITER-1/MATLAB Function1 ==
  data: VT input; u output; QT input; PT input
function u = fcn(VT,QT,PT)
Xq=0.474;
Kadj= (((VT*VT)/Xq)+QT)/(sqrt(((((VT*VT)/Xq)+QT)*(((VT*VT)/Xq)+QT))+(PT*PT)))
u= Kadj;

== matlab function SSN_39busRT_Ctrl_4WT_19B/SM_master/G4/G4/ST6C EXCITER-1/MATLAB Function2 ==
  data: ISCLERR input; IOEX2 output; ISCLINV input; IUEX2 output
function [IOEX2,IUEX2] = fcn(ISCLERR,ISCLINV)
%#codegen

IOEX2= 0;
IUEX2= 0;

== matlab function SSN_39busRT_Ctrl_4WT_19B/SM_master/G7/G7/ST6C EXCITER-1/MATLAB Function ==
  data: VTF input; u output; Vbias input
function u = fcn(VTF,Vbias)
%#codegen
if VTF > 1
    u=VTF;
    
else if VTF > Vbias
        u=1;
    else
        u=VTF/Vbias
    end
end
u;

== matlab function SSN_39busRT_Ctrl_4WT_19B/SM_master/G7/G7/ST6C EXCITER-1/MATLAB Function1 ==
  data: VT input; u output; QT input; PT input
function u = fcn(VT,QT,PT)
Xq=0.474;
Kadj= (((VT*VT)/Xq)+QT)/(sqrt(((((VT*VT)/Xq)+QT)*(((VT*VT)/Xq)+QT))+(PT*PT)))
u= Kadj;

== matlab function SSN_39busRT_Ctrl_4WT_19B/SM_master/G7/G7/ST6C EXCITER-1/MATLAB Function2 ==
  data: ISCLERR input; IOEX2 output; ISCLINV input; IUEX2 output
function [IOEX2,IUEX2] = fcn(ISCLERR,ISCLINV)
%#codegen

IOEX2= 0;
IUEX2= 0;

== matlab function SSN_39busRT_Ctrl_4WT_19B/SM_master/G3/G3/ST6C EXCITER-1/MATLAB Function ==
  data: VTF input; u output; Vbias input
function u = fcn(VTF,Vbias)
%#codegen
if VTF > 1
    u=VTF;
    
else if VTF > Vbias
        u=1;
    else
        u=VTF/Vbias
    end
end
u;

== matlab function SSN_39busRT_Ctrl_4WT_19B/SM_master/G3/G3/ST6C EXCITER-1/MATLAB Function1 ==
  data: VT input; u output; QT input; PT input
function u = fcn(VT,QT,PT)
Xq=0.474;
Kadj= (((VT*VT)/Xq)+QT)/(sqrt(((((VT*VT)/Xq)+QT)*(((VT*VT)/Xq)+QT))+(PT*PT)))
u= Kadj;

== matlab function SSN_39busRT_Ctrl_4WT_19B/SM_master/G3/G3/ST6C EXCITER-1/MATLAB Function2 ==
  data: ISCLERR input; IOEX2 output; ISCLINV input; IUEX2 output
function [IOEX2,IUEX2] = fcn(ISCLERR,ISCLINV)
%#codegen

IOEX2= 0;
IUEX2= 0;

== matlab function SSN_39busRT_Ctrl_4WT_19B/SM_master/G10/G10/ST6C EXCITER-1/MATLAB Function2 ==
  data: ISCLERR input; IOEX2 output; ISCLINV input; IUEX2 output
function [IOEX2,IUEX2] = fcn(ISCLERR,ISCLINV)
%#codegen

IOEX2= 0;
IUEX2= 0;

== matlab function SSN_39busRT_Ctrl_4WT_19B/SM_master/G9/G9/ST6C EXCITER-1/MATLAB Function ==
  data: VTF input; u output; Vbias input
function u = fcn(VTF,Vbias)
%#codegen
if VTF > 1
    u=VTF;
    
else if VTF > Vbias
        u=1;
    else
        u=VTF/Vbias
    end
end
u;

== matlab function SSN_39busRT_Ctrl_4WT_19B/SM_master/G9/G9/ST6C EXCITER-1/MATLAB Function1 ==
  data: VT input; u output; QT input; PT input
function u = fcn(VT,QT,PT)
Xq=0.474;
Kadj= (((VT*VT)/Xq)+QT)/(sqrt(((((VT*VT)/Xq)+QT)*(((VT*VT)/Xq)+QT))+(PT*PT)))
u= Kadj;

== matlab function SSN_39busRT_Ctrl_4WT_19B/SM_master/G9/G9/ST6C EXCITER-1/MATLAB Function2 ==
  data: ISCLERR input; IOEX2 output; ISCLINV input; IUEX2 output
function [IOEX2,IUEX2] = fcn(ISCLERR,ISCLINV)
%#codegen

IOEX2= 0;
IUEX2= 0;

== matlab function SSN_39busRT_Ctrl_4WT_19B/SM_master/G1/G1/ST6C EXCITER-1/MATLAB Function ==
  data: VTF input; u output; Vbias input
function u = fcn(VTF,Vbias)
%#codegen
if VTF > 1
    u=VTF;
    
else if VTF > Vbias
        u=1;
    else
        u=VTF/Vbias
    end
end
u;

== matlab function SSN_39busRT_Ctrl_4WT_19B/SM_master/G1/G1/ST6C EXCITER-1/MATLAB Function1 ==
  data: VT input; u output; QT input; PT input
function u = fcn(VT,QT,PT)
Xq=0.474;
Kadj= (((VT*VT)/Xq)+QT)/(sqrt(((((VT*VT)/Xq)+QT)*(((VT*VT)/Xq)+QT))+(PT*PT)))
u= Kadj;

== matlab function SSN_39busRT_Ctrl_4WT_19B/SM_master/G1/G1/ST6C EXCITER-1/MATLAB Function2 ==
  data: ISCLERR input; IOEX2 output; ISCLINV input; IUEX2 output
function [IOEX2,IUEX2] = fcn(ISCLERR,ISCLINV)
%#codegen

IOEX2= 0;
IUEX2= 0;

== matlab function SSN_39busRT_Ctrl_4WT_19B/SM_master/G2/G2/ST6C EXCITER-1/MATLAB Function ==
  data: VTF input; u output; Vbias input
function u = fcn(VTF,Vbias)
%#codegen
if VTF > 1
    u=VTF;
    
else if VTF > Vbias
        u=1;
    else
        u=VTF/Vbias
    end
end
u;

== matlab function SSN_39busRT_Ctrl_4WT_19B/SM_master/G8/ G8/ST6C EXCITER-1/MATLAB Function ==
  data: VTF input; u output; Vbias input
function u = fcn(VTF,Vbias)
%#codegen
if VTF > 1
    u=VTF;
    
else if VTF > Vbias
        u=1;
    else
        u=VTF/Vbias
    end
end
u;
